simulink model "generatorfull"  (Simulink 8.4)
settings: Solver=ode15s  StartTime=0.0  StopTime=110  RelTol=1e-3
values from neighbouring files (symbols this model uses):
  AvrSat = 20*sqrt(2/3)    [articlerun.m]
  DataSamplingTime = T(end)/Datapoints    [articlerun.m]
  Davr = 0    [articlerun.m]
  Dgovernor = 10    [articlerun.m]
  droopAVR = 0.05    [articlerun.m]    (also in m1.m)
  droopGovernor = 0    [articlerun.m]    (also in m1.m)
  H = 5.6    [articlerun.m]    (also in m1.m = 0.5*J_rotor*wbasem*wbasem/Sbase)
  Iavr = 0    [articlerun.m]
  Igovernor = 10    [articlerun.m]
  Ki = [-1/Xls 0       0       0       0       0       1/Xls   0 ... (first row only)    [articlerun.m]    (also in m1.m)
  Kmqmd = [ Xaq/Xls 0     0   Xaq/Xlkq2   0       0 ... (first row only)    [articlerun.m]    (also in m1.m = [ Xaq/Xls 0     0   Xaq/Xlkq2 0       0)
  Kpsi = [-rs/Xls 0     0       0       0       0       rs/Xls  0 ... (first row only)    [articlerun.m]    (also in m1.m = wb*Kpsi)
  Kv = [  1       0       0       0       0       0 ... (first row only)    [articlerun.m]    (also in m1.m = wb*Kv)
  Kwpsi = [0 -1   0   0   0   0 ... (first row only)    [articlerun.m]    (also in m1.m = zeros(6))
  loadAmplitude = 0    [initArt.m]
  loadBias = 0.5    [initArt.m]
  loadfreq = 2*pi/loadT    (= 628.318530718)    [initArt.m]
  loadStep = 0    [initArt.m]
  loadStepTime = 15    [initArt.m]
  Pavr = 400    [articlerun.m]
  Pgovernor = 20    [articlerun.m]
  psiInit = Psi.signals.values(end,1:7)    [articlerun.m]    (also in init.mat = [-391.464820784 14501.79303 -1.35791716672e-12 -350.14204148; m1.m = psiInit([1 2 3 5 6 7]))
  ShortCircuitOn = 0    [articlerun.m]    (also in m1.m)
  ShortCircuitStart = 0    [articlerun.m]    (also in m1.m)
  ShortCircuitStop = 0    [articlerun.m]    (also in m1.m)
  thetaInit = theta(end)*pi/180    [articlerun.m]    (also in init.mat = 0.0269876819053)
  wb = 60*2*pi    (= 376.991118431)    [articlerun.m]    (also in m1.m)
libraries: simulink x3
settings Model: Creator=tibnor  LastModifiedBy=torsteinibo
settings DataIOCC: InspectSignalLogs=on

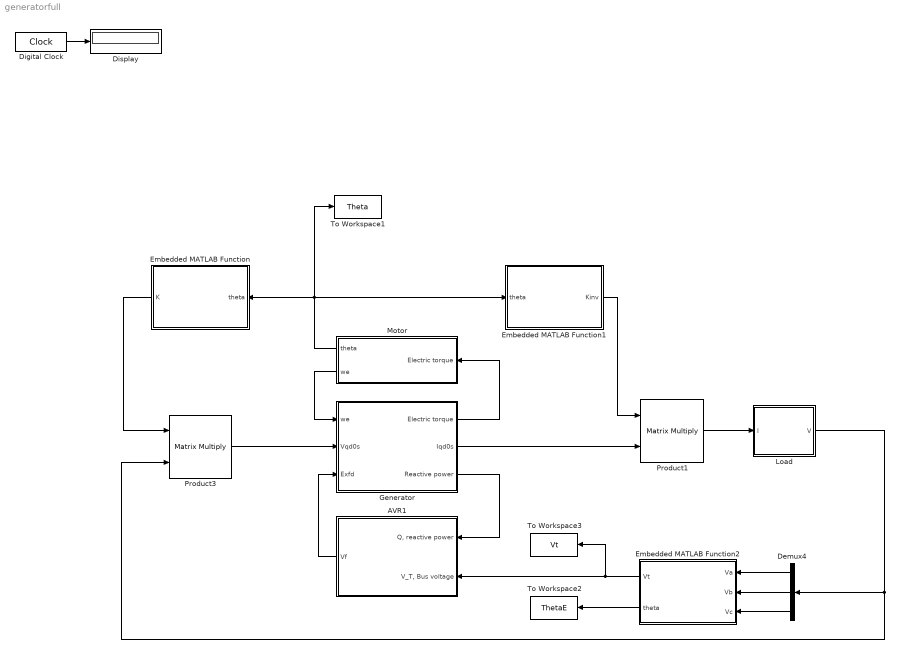
== system generatorfull ==
  AVR1 : Subsystem  AncestorBlock=PMSlib/Genset/AVR
  Demux4 : Demux  Outputs=3
  Digital Clock : DigitalClock  SampleTime=DataSamplingTime
  Display : Display
  Embedded MATLAB Function : MATLAB Function  TreatAsAtomicUnit=on
  Embedded MATLAB Function1 : MATLAB Function  TreatAsAtomicUnit=on
  Embedded MATLAB Function2 : MATLAB Function  TreatAsAtomicUnit=on
  Generator : Subsystem
  Load : Subsystem
  Motor : Subsystem
  Product1 : Product  Multiplication=Matrix(*)  RndMeth=Zero
  Product3 : Product  Multiplication=Matrix(*)  RndMeth=Zero
  To Workspace1 : ToWorkspace  VariableName=Theta  SaveFormat=Structure With Time  SampleTime=DataSamplingTime
  To Workspace2 : ToWorkspace  VariableName=ThetaE  SaveFormat=Structure With Time  SampleTime=DataSamplingTime
  To Workspace3 : ToWorkspace  VariableName=Vt  SaveFormat=Structure With Time  SampleTime=DataSamplingTime
  wires:
  Embedded MATLAB Function/1(K) -> Product3/1
  Product3/1 -> Generator/2(Vqd0s)
  Digital Clock/1 -> Display/1
  Generator/3(Reactive power) -> AVR1/1("Q, reactive power")
  Generator/1(Electric torque) -> Motor/1(Electric torque)
  Motor/2(we) -> Generator/1(we)
  Generator/2(Iqd0s) -> Product1/2
  Motor/1(theta) -> To Workspace1/1, Embedded MATLAB Function1/1(theta), Embedded MATLAB Function/1(theta)
  Embedded MATLAB Function1/1(Kinv) -> Product1/1
  Product1/1 -> Load/1(I)
  Load/1(V) -> Product3/2, Demux4/1
  Embedded MATLAB Function2/1(Vt) -> AVR1/2("V_T, Bus voltage"), To Workspace3/1
  AVR1/1(Vf) -> Generator/3(Exfd)
  Demux4/1 -> Embedded MATLAB Function2/1(Va)
  Demux4/2 -> Embedded MATLAB Function2/2(Vb)
  Demux4/3 -> Embedded MATLAB Function2/3(Vc)
  Embedded MATLAB Function2/2(theta) -> To Workspace2/1

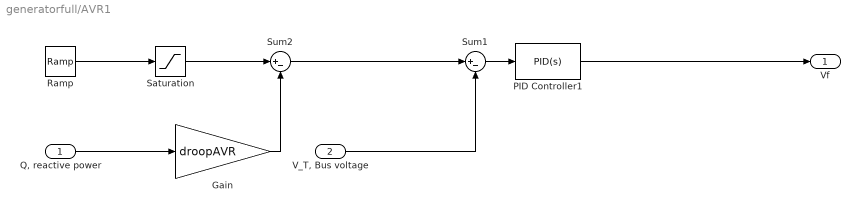
== system generatorfull/AVR1 ==
  "Q, reactive power" : Inport
  "V_T, Bus voltage" : Inport  Port=2
  Gain : Gain  Gain=droopAVR
  PID Controller1 : simulink/Continuous/PID Controller  Controller=PID  TimeDomain=Continuous-time  SampleTime=-1  IntegratorMethod=Forward Euler  FilterMethod=Forward Euler  Form=Parallel  P=Pavr  I=Iavr  D=Davr  N=100  InitialConditionSource=internal  InitialConditionForIntegrator=exfdo  InitialConditionForFilter=0  ExternalReset=none  LimitOutput=on  UpperSaturationLimit=AvrSat  LowerSaturationLimit=-AvrSat  LinearizeAsGain=off  AntiWindupMode=none  Kb=1  TrackingMode=off  Kt=1  PParamMin=[]  PParamMax=[]  IParamMin=[]  IParamMax=[]  DParamMin=[]  DParamMax=[]  NParamMin=[]  NParamMax=[]  KbParamMin=[]  KbParamMax=[]  KtParamMin=[]  KtParamMax=[]  POutMin=[]  POutMax=[]  IOutMin=[]  IOutMax=[]  DOutMin=[]  DOutMax=[]  NOutMin=[]  NOutMax=[]  KbOutMin=[]  KbOutMax=[]  KtOutMin=[]  KtOutMax=[]  IntegratorOutMin=[]  IntegratorOutMax=[]  FilterOutMin=[]  FilterOutMax=[]  SumOutMin=[]  SumOutMax=[]  SumI1OutMin=[]  SumI1OutMax=[]  SumI2OutMin=[]  SumI2OutMax=[]  SumI3OutMin=[]  SumI3OutMax=[]  SumDOutMin=[]  SumDOutMax=[]  SaturationOutMin=[]  SaturationOutMax=[]  IntegratorContinuousStateAttributes=''  IntegratorStateMustResolveToSignalObject=off  IntegratorRTWStateStorageClass=Auto  FilterContinuousStateAttributes=''  FilterStateMustResolveToSignalObject=off  FilterRTWStateStorageClass=Auto  DifferentiatorICPrevScaledInput=0  DifferentiatorOutMin=[]  DifferentiatorOutMax=[]  UseFilter=on
  Ramp : simulink/Sources/Ramp  slope=1/100  start=0  X0=0
  Saturation : Saturate  UpperLimit=1  LowerLimit=0
  Sum1 : Sum  Inputs=|+-
  Sum2 : Sum  Inputs=|+-
  Vf : Outport
  wires:
  Gain/1 -> Sum2/2
  Sum2/1 -> Sum1/1
  Ramp/1 -> Saturation/1
  Sum1/1 -> PID Controller1/1
  "Q, reactive power"/1 -> Gain/1
  "V_T, Bus voltage"/1 -> Sum1/2
  PID Controller1/1 -> Vf/1
  Saturation/1 -> Sum2/1

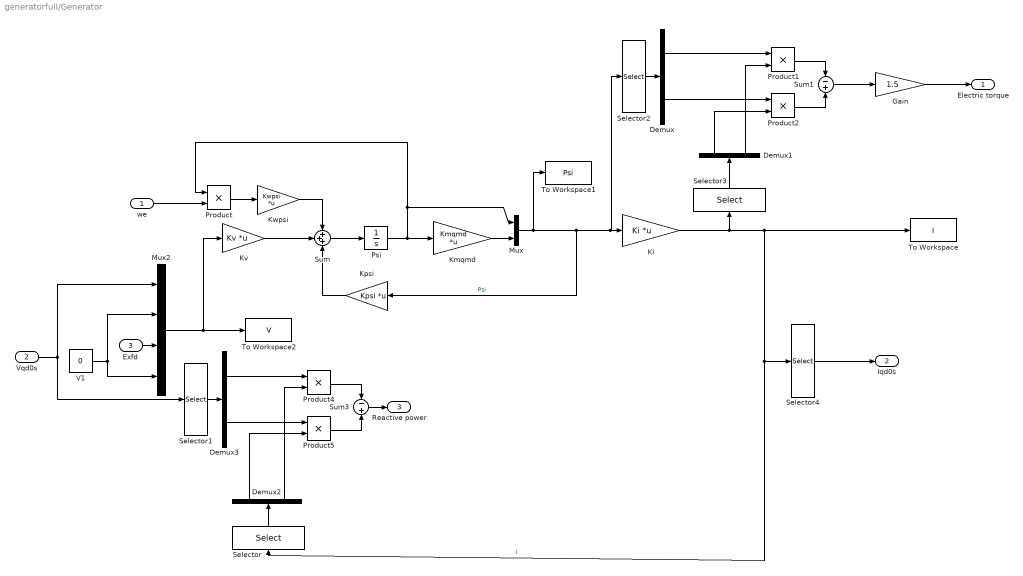
== system generatorfull/Generator ==
  we : Inport
  Vqd0s : Inport  Port=2
  Exfd : Inport  Port=3
  Demux{,1..3} (4 alike) : Demux  Outputs=2
  Gain : Gain  Gain=1.5
  Ki : Gain  Gain=Ki  Multiplication=Matrix(K*u)
  Kmqmd : Gain  Gain=Kmqmd  Multiplication=Matrix(K*u)
  Kpsi : Gain  Gain=Kpsi  Multiplication=Matrix(K*u)
  Kv : Gain  Gain=Kv  Multiplication=Matrix(K*u)
  Kwpsi : Gain  Gain=Kwpsi  Multiplication=Matrix(K*u)
  Mux : Mux  Inputs=2
  Mux2 : Mux
  Product{,1..2,4..5} (5 alike) : Product  RndMeth=Zero
  Psi : Integrator  InitialCondition=psiInit
  Selector : Selector  InputPortWidth=6  Indices=[1 2]
  Selector1 : Selector  InputPortWidth=3  Indices=[1 2]
  Selector2 : Selector  InputPortWidth=8  Indices=[1 2]
  Selector3 : Selector  InputPortWidth=6  Indices=[1 2]
  Selector4 : Selector  InputPortWidth=6  Indices=[1 2 3]
  Sum : Sum  Inputs=+++
  Sum1 : Sum  Inputs=-+
  Sum3 : Sum  Inputs=-+
  To Workspace : ToWorkspace  VariableName=I  SaveFormat=Structure With Time  SampleTime=DataSamplingTime
  To Workspace1 : ToWorkspace  VariableName=Psi  SaveFormat=Structure With Time  SampleTime=DataSamplingTime
  To Workspace2 : ToWorkspace  VariableName=V  SaveFormat=Structure With Time  SampleTime=DataSamplingTime
  V1 : Constant  Value=0
  Electric torque : Outport
  Iqd0s : Outport  Port=2
  Reactive power : Outport  Port=3
  wires:
  Psi/1 -> Kmqmd/1, Mux/1, Product/1
  Sum/1 -> Psi/1
  Product/1 -> Kwpsi/1
  Kwpsi/1 -> Sum/1
  Kv/1 -> Sum/2
  Kpsi/1 -> Sum/3
  Kmqmd/1 -> Mux/2
  Mux/1 -> Kpsi/1, Selector2/1, Ki/1, To Workspace1/1  "Psi"
  Ki/1 -> To Workspace/1, Selector4/1, Selector/1, Selector3/1  "I"
  Demux1/2 -> Product1/2
  Demux/1 -> Product1/1
  Demux/2 -> Product2/1
  Demux1/1 -> Product2/2
  Product2/1 -> Sum1/2
  Product1/1 -> Sum1/1
  Mux2/1 -> Kv/1, To Workspace2/1
  Product5/1 -> Sum3/2
  Product4/1 -> Sum3/1
  Demux3/1 -> Product4/1
  Demux2/2 -> Product4/2
  V1/1 -> Mux2/4, Mux2/2
  we/1 -> Product/2
  Vqd0s/1 -> Selector1/1, Mux2/1
  Exfd/1 -> Mux2/3
  Sum1/1 -> Gain/1
  Sum3/1 -> Reactive power/1
  Demux3/2 -> Product5/1
  Demux2/1 -> Product5/2
  Gain/1 -> Electric torque/1
  Selector/1 -> Demux2/1
  Selector1/1 -> Demux3/1
  Selector2/1 -> Demux/1
  Selector3/1 -> Demux1/1
  Selector4/1 -> Iqd0s/1

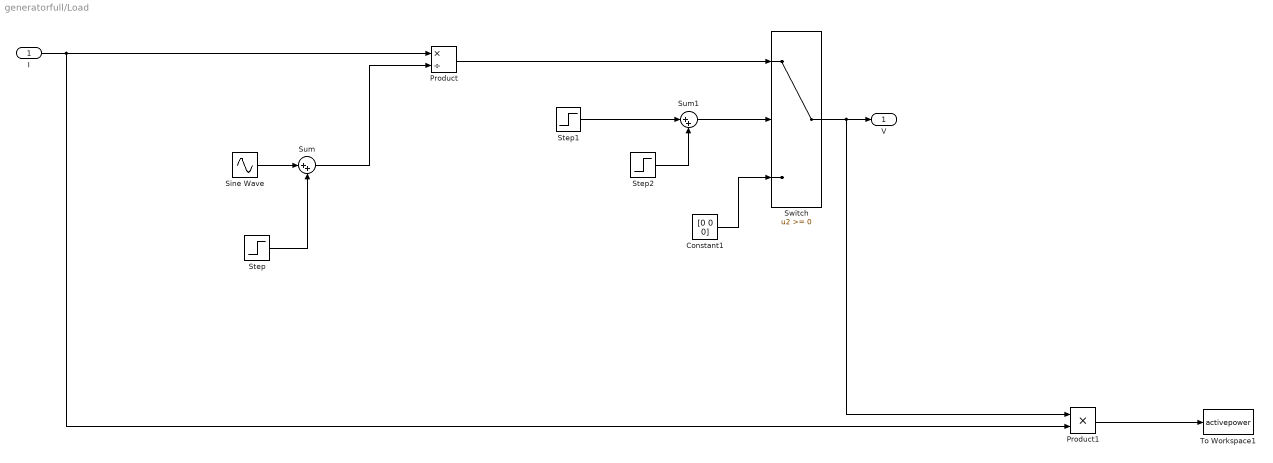
== system generatorfull/Load ==
  I : Inport
  Constant1 : Constant  Value=[0 0 0]
  Product : Product  Inputs=*/  RndMeth=Zero
  Product1 : Product  RndMeth=Zero
  Sine Wave : Sin  Amplitude=loadAmplitude  Bias=loadBias  Frequency=loadfreq  SampleTime=0
  Step : Step  Time=loadStepTime  After=loadStep  SampleTime=0
  Step1 : Step  Time=ShortCircuitStart  After=-ShortCircuitOn  SampleTime=0
  Step2 : Step  Time=ShortCircuitStop  After=ShortCircuitOn  SampleTime=0
  Sum : Sum  Inputs=|++
  Sum1 : Sum  Inputs=|++
  Switch : Switch
  To Workspace1 : ToWorkspace  VariableName=activepower  SaveFormat=Structure With Time  SampleTime=DataSamplingTime
  V : Outport
  wires:
  I/1 -> Product/1, Product1/2
  Sine Wave/1 -> Sum/1
  Sum/1 -> Product/2
  Step/1 -> Sum/2
  Product/1 -> Switch/1
  Sum1/1 -> Switch/2
  Step1/1 -> Sum1/1
  Step2/1 -> Sum1/2
  Constant1/1 -> Switch/3
  Switch/1 -> V/1, Product1/1
  Product1/1 -> To Workspace1/1

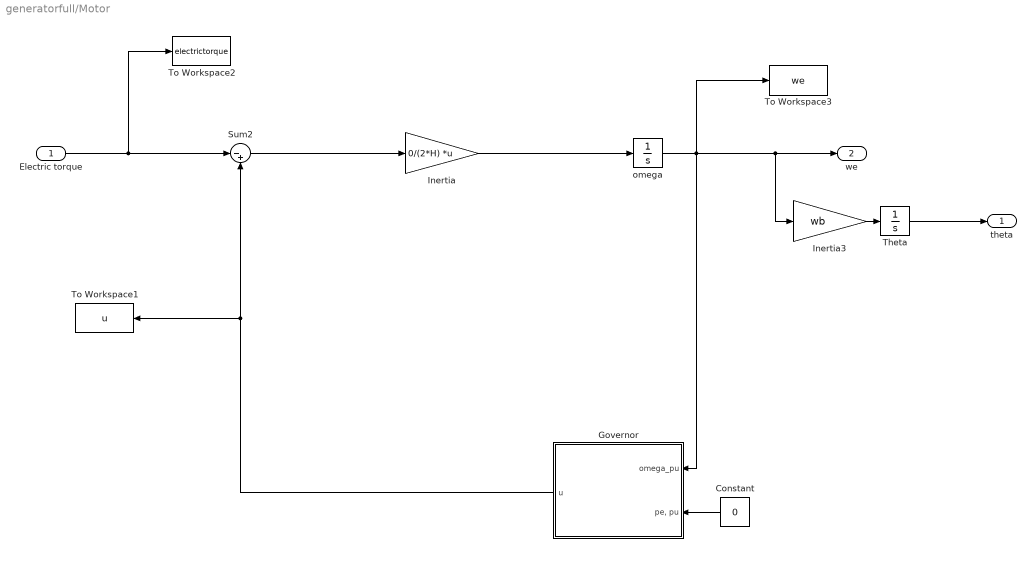
== system generatorfull/Motor ==
  Electric torque : Inport
  Constant : Constant  Value=0
  Governor : Subsystem  AncestorBlock=PMSlib/Genset/Governor
  Inertia : Gain  Gain=0/(2*H)  Multiplication=Matrix(K*u)
  Inertia3 : Gain  Gain=wb
  Sum2 : Sum  Inputs=|-+
  Theta : Integrator  InitialCondition=thetaInit
  To Workspace1 : ToWorkspace  VariableName=u  SaveFormat=Structure With Time  SampleTime=DataSamplingTime
  To Workspace2 : ToWorkspace  VariableName=electrictorque  SaveFormat=Structure With Time  SampleTime=DataSamplingTime
  To Workspace3 : ToWorkspace  VariableName=we  SaveFormat=Structure With Time  SampleTime=DataSamplingTime
  omega : Integrator  InitialCondition=1
  theta : Outport
  we : Outport  Port=2
  wires:
  Sum2/1 -> Inertia/1
  Inertia/1 -> omega/1
  Electric torque/1 -> To Workspace2/1, Sum2/1
  omega/1 -> Governor/1(omega_pu), Inertia3/1, we/1, To Workspace3/1
  Constant/1 -> Governor/2("pe, pu")
  Governor/1(u) -> To Workspace1/1, Sum2/2
  Inertia3/1 -> Theta/1
  Theta/1 -> theta/1

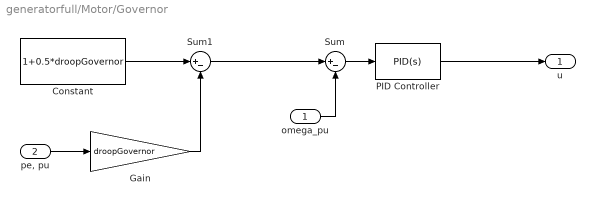
== system generatorfull/Motor/Governor ==
  omega_pu : Inport
  "pe, pu" : Inport  Port=2
  Constant : Constant  Value=1+0.5*droopGovernor
  Gain : Gain  Gain=droopGovernor
  PID Controller : simulink/Continuous/PID Controller  Controller=PID  TimeDomain=Continuous-time  SampleTime=-1  IntegratorMethod=Forward Euler  FilterMethod=Forward Euler  Form=Parallel  P=Pgovernor  I=Igovernor  D=Dgovernor  N=100  InitialConditionSource=internal  InitialConditionForIntegrator=0  InitialConditionForFilter=0  ExternalReset=none  LimitOutput=on  UpperSaturationLimit=2  LowerSaturationLimit=0  LinearizeAsGain=off  AntiWindupMode=none  Kb=1  TrackingMode=off  Kt=1  PParamMin=[]  PParamMax=[]  IParamMin=[]  IParamMax=[]  DParamMin=[]  DParamMax=[]  NParamMin=[]  NParamMax=[]  KbParamMin=[]  KbParamMax=[]  KtParamMin=[]  KtParamMax=[]  POutMin=[]  POutMax=[]  IOutMin=[]  IOutMax=[]  DOutMin=[]  DOutMax=[]  NOutMin=[]  NOutMax=[]  KbOutMin=[]  KbOutMax=[]  KtOutMin=[]  KtOutMax=[]  IntegratorOutMin=[]  IntegratorOutMax=[]  FilterOutMin=[]  FilterOutMax=[]  SumOutMin=[]  SumOutMax=[]  SumI1OutMin=[]  SumI1OutMax=[]  SumI2OutMin=[]  SumI2OutMax=[]  SumI3OutMin=[]  SumI3OutMax=[]  SumDOutMin=[]  SumDOutMax=[]  SaturationOutMin=[]  SaturationOutMax=[]  IntegratorContinuousStateAttributes=''  IntegratorStateMustResolveToSignalObject=off  IntegratorRTWStateStorageClass=Auto  FilterContinuousStateAttributes=''  FilterStateMustResolveToSignalObject=off  FilterRTWStateStorageClass=Auto  DifferentiatorICPrevScaledInput=0  DifferentiatorOutMin=[]  DifferentiatorOutMax=[]  UseFilter=on
  Sum : Sum  Inputs=|+-
  Sum1 : Sum  Inputs=|+-
  u : Outport
  wires:
  Gain/1 -> Sum1/2
  "pe, pu"/1 -> Gain/1
  Sum1/1 -> Sum/1
  Constant/1 -> Sum1/1
  omega_pu/1 -> Sum/2
  Sum/1 -> PID Controller/1
  PID Controller/1 -> u/1

== matlab function Embedded MATLAB Function1 ==
  data: theta input double; Kinv output double
function Kinv = RotationInv(theta)

Kinv = [cos(theta)         sin(theta)      1
     cos(theta-2*pi/3)  sin(theta-2*pi/3)   1
     cos(theta+2*pi/3)  sin(theta+2*pi/3)   1];

== matlab function Embedded MATLAB Function ==
  data: theta input double; K output double
function K = Rotation(theta)

K = 2/3*[cos(theta) cos(theta-2*pi/3) cos(theta+2*pi/3)
         sin(theta) sin(theta-2*pi/3) sin(theta+2*pi/3)
         .5         .5                 .5];

== matlab function Embedded MATLAB Function2 ==
  data: Va input double; Vt output double; Vb input double; Vc input double; theta output double
function [Vt,theta] = LengthV(Va, Vb, Vc)

Vb = Vb*exp(2/3*pi*1j);
Vc = Vc*exp(-2/3*pi*1j);

V = Va+Vb+Vc;

Vt = abs(V)*sqrt(2/3);
theta = angle(V);
